simulink model "inverted_pendulum_linear_model"  (R2021a)
settings: Solver=ode4  StartTime=0.0  StopTime=tEnd  FixedStep=dt  RelTol=1e-3
values from neighbouring files (symbols this model uses):
  A = [0      1                   0                           0 ... (first row only)    [inv_pend_SS.m]
  B = [0 ... (first row only)    [inv_pend_SS.m]
  C = eye(4)    [inv_pend_SS.m]
  D = [0;0;0;0]    [inv_pend_SS.m]
  K = lqr(sys,Q,R)    [QR_Optimization.m]    (also in main.m = K_LQR .* 0)
  thetaMax = 100 * DTOR    (= 1.74532925199)    [main.m]
  x0 = initWeights    [QR_Optimization.m]    (also in createScenario.m = [0 0 1 0]; main.m = [0 0 .01 0])
settings Model: PacingRate=0.110000  Creator=Jeff  LastModifiedBy=jordan
settings SolverCC: AlgebraicLoopSolver=TrustRegion
settings DebuggingCC: SFMachineParentedDataDiag=warning  ArithmeticOperatorsInVariantConditions=warning
settings SFSimCC: CustomCodeUndefinedFunction=UseInterfaceOnly

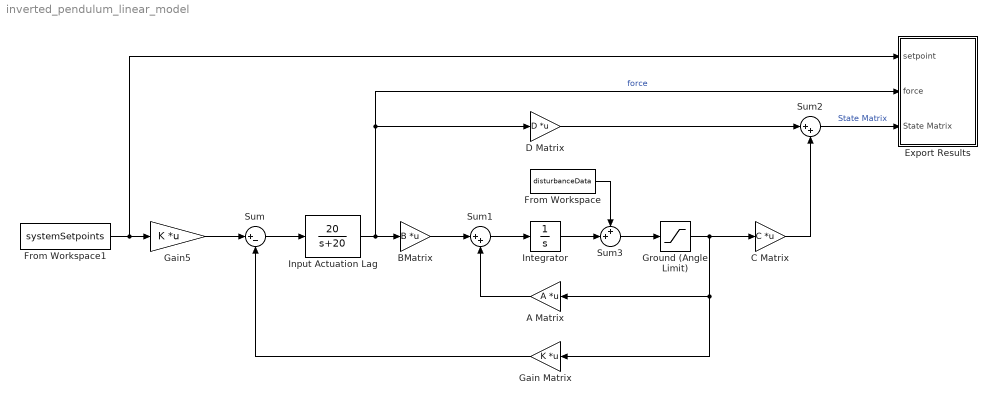
== system inverted_pendulum_linear_model ==
  A Matrix : Gain  Gain=A  Multiplication=Matrix(K*u)
  BMatrix : Gain  Gain=B  Multiplication=Matrix(K*u)
  C Matrix : Gain  Gain=C  Multiplication=Matrix(K*u)
  D Matrix : Gain  Gain=D  Multiplication=Matrix(K*u)
  Export Results : Subsystem
  From Workspace : FromWorkspace  VariableName=disturbanceData
  From Workspace1 : FromWorkspace  VariableName=systemSetpoints
  Gain Matrix : Gain  Gain=K  Multiplication=Matrix(K*u)
  Gain5 : Gain  Gain=K  Multiplication=Matrix(K*u)
  Ground (Angle Limit) : Saturate  UpperLimit=[10^6 10^6 thetaMax 10^6]  LowerLimit=-[10^6 10^6 thetaMax 10^6]
  Input Actuation Lag : TransferFcn  Numerator=[20]  Denominator=[1 20]
  Integrator : Integrator  InitialCondition=x0
  Sum : Sum  Inputs=|+-
  Sum1 : Sum  Inputs=|++
  Sum2 : Sum  Inputs=|++
  Sum3 : Sum  Inputs=++|
  wires:
  Integrator/1 -> Sum3/2
  Sum3/1 -> Ground (Angle Limit)/1
  Ground (Angle Limit)/1 -> C Matrix/1, A Matrix/1, Gain Matrix/1
  Sum/1 -> Input Actuation Lag/1
  From Workspace/1 -> Sum3/1
  Input Actuation Lag/1 -> Export Results/2(force), D Matrix/1, BMatrix/1  "force"
  From Workspace1/1 -> Export Results/1(setpoint), Gain5/1
  Gain5/1 -> Sum/1
  Gain Matrix/1 -> Sum/2
  C Matrix/1 -> Sum2/2
  Sum1/1 -> Integrator/1
  A Matrix/1 -> Sum1/2
  BMatrix/1 -> Sum1/1
  D Matrix/1 -> Sum2/1
  Sum2/1 -> Export Results/3(State Matrix)  "State Matrix"

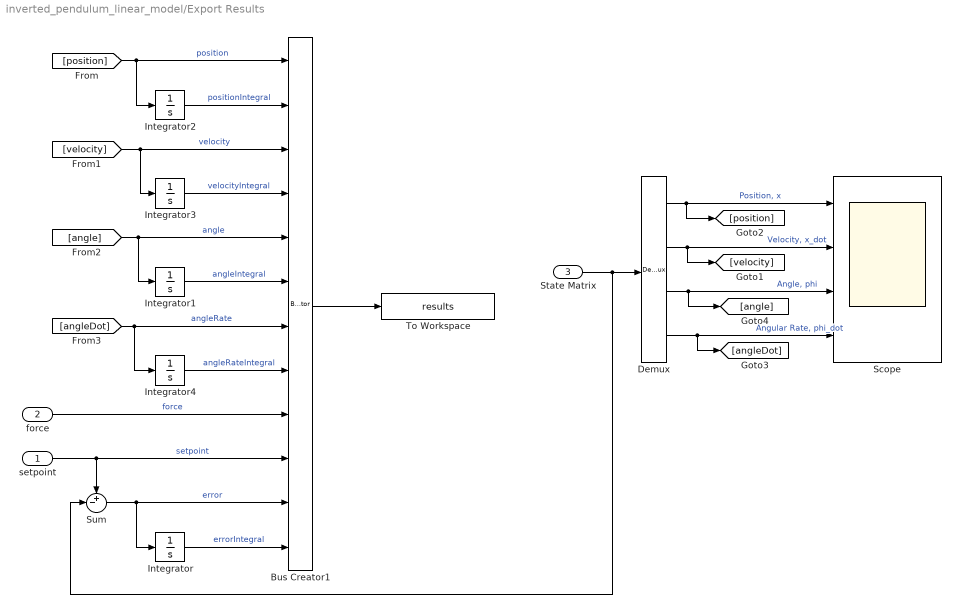
== system inverted_pendulum_linear_model/Export Results ==
  setpoint : Inport
  force : Inport  Port=2
  State Matrix : Inport  Port=3
  Bus Creator1 : BusCreator  Inputs=12
  Demux : Demux
  Integrator{,1..4} (5 alike) : Integrator
  Scope : Scope  NumInputPorts=4
  Sum : Sum  Inputs=+-|
  To Workspace : ToWorkspace  VariableName=results  SaveFormat=Timeseries  SampleTime=-1
  wires:
  [position] -> Integrator2/1, Bus Creator1/1  "position"
  Demux/3 -> [angle], Scope/3  "Angle, phi"
  [velocity] -> Integrator3/1, Bus Creator1/3  "velocity"
  Demux/2 -> [velocity], Scope/2  "Velocity, x_dot"
  Integrator4/1 -> Bus Creator1/8  "angleRateIntegral"
  Demux/1 -> Scope/1, [position]  "Position, x"
  Bus Creator1/1 -> To Workspace/1
  Demux/4 -> Scope/4, [angleDot]  "Angular Rate, phi_dot"
  [angle] -> Integrator1/1, Bus Creator1/5  "angle"
  [angleDot] -> Integrator4/1, Bus Creator1/7  "angleRate"
  Integrator2/1 -> Bus Creator1/2  "positionIntegral"
  Integrator1/1 -> Bus Creator1/6  "angleIntegral"
  Integrator3/1 -> Bus Creator1/4  "velocityIntegral"
  force/1 -> Bus Creator1/9  "force"
  State Matrix/1 -> Sum/2, Demux/1
  Sum/1 -> Integrator/1, Bus Creator1/11  "error"
  Integrator/1 -> Bus Creator1/12  "errorIntegral"
  setpoint/1 -> Bus Creator1/10, Sum/1  "setpoint"
